simulink model "Output_Feedback_Teleoperation"  (Simulink 8.6)
settings: Solver=ode45  StartTime=0.0  StopTime=40  FixedStep=0.001  RelTol=1e-3
values from neighbouring files (symbols this model uses):
  c1 = 5    [Parameters.m]
  c2 = 5    [Parameters.m]
  c3 = 5    [Parameters.m]
  l1 = Prm(3)    [Coriolis.m]    (also in Inertia.m; P1.m; P2.m; Parameters.m = 0.4)
  l2 = Prm(4)    [Coriolis.m]    (also in Inertia.m; P1.m; P2.m; Parameters.m = 0.3)
  q_dot0 = [0;0]    [Parameters.m]
  q_hat0 = [0;0]    [Parameters.m]
  r_0 = 0    [Parameters.m]
  x_hat0 = [0;0]    [Parameters.m]
  xi_0 = [0;0]    [Parameters.m]
undefined symbols (not defined in the file or in its folder): cr, dm, ds, Kd, Kh, kl, kr, ml1, ml2, mr1, mr2, pl, pr, Pwall, ql_0, qr_0, sigbuilder_block
libraries: simulink x1
settings Model: Creator=TOSHIBA  LastModifiedBy=TOSHIBA
settings DataIOCC: SaveFormat=StructureWithTime  SignalLoggingSaveFormat=Dataset
settings OptimizationCC: ExpressionDepthLimit=128
settings DebuggingCC: UnderspecifiedInitializationDetection=Simplified  MergeDetectMultiDrivingBlocksExec=error  SolverPrmCheckMsg=none  FcnCallInpInsideContextMsg=EnableAllAsError  StateNameClashWarn=none
settings HardwareCC: ProdBitPerPointer=64  ProdLargestAtomicFloat=Float  ProdIntDivRoundTo=Zero  ProdEndianess=LittleEndian  ProdHWDeviceType=Specified
settings GRTTargetCC: GeneratePreprocessorConditionals=Use local settings  CombineOutputUpdateFcns=on  GRTInterface=off
settings ConfigComp: CovModelRefEnable=off

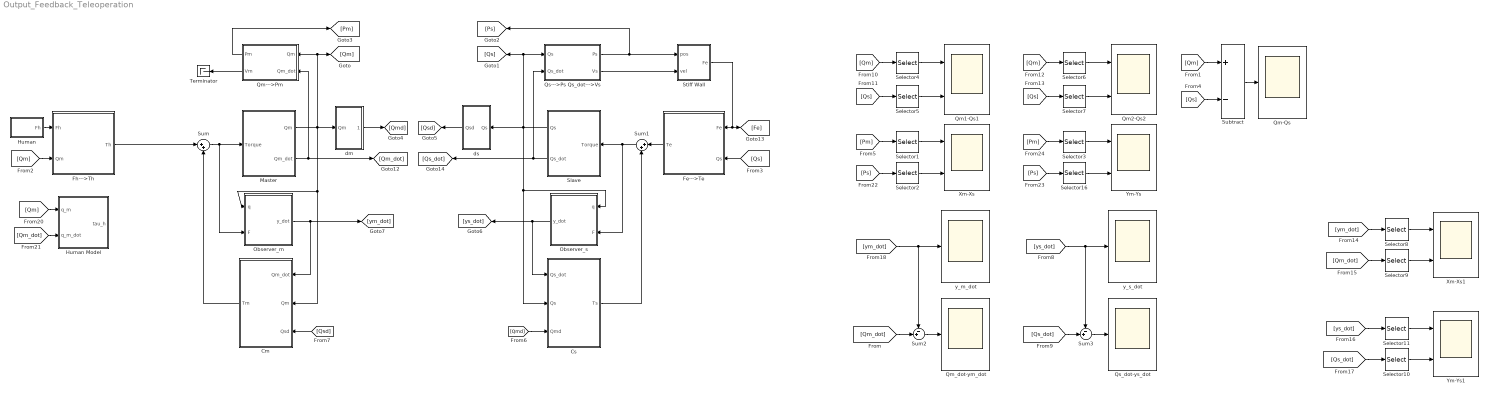
== system Output_Feedback_Teleoperation ==
  Cm : Subsystem
  Cs : Subsystem
  Fe--->Te : Subsystem
  Fh--->Th : Subsystem
  Human : Subsystem
  Human Model : Subsystem
  Master : Subsystem
  Observer_m : Subsystem
  Observer_s : Subsystem
  Qm--->Pm : Subsystem
  Qm-Qs : Scope
  Qm1-Qs1 : Scope  NumInputPorts=2
  Qm2-Qs2 : Scope  NumInputPorts=2
  Qm_dot-ym_dot : Scope
  Qs--->Ps Qs_dot--->Vs : Subsystem
  Qs_dot-ys_dot : Scope
  Selector{1..2,4..5,8..11} (8 alike) : Selector  InputPortWidth=2  IndexOptions=Index vector (dialog)  Indices=[1]  OutputSizes=1
  Selector{3,6..7,16} (4 alike) : Selector  InputPortWidth=2  IndexOptions=Index vector (dialog)  Indices=[2]  OutputSizes=1
  Slave : Subsystem
  Stiff Wall : Subsystem
  Subtract : Sum  Inputs=+-
  Sum : Sum  Inputs=|++
  Sum1 : Sum  Inputs=|++
  Sum2 : Sum  Inputs=-+|
  Sum3 : Sum  Inputs=-+|
  Terminator : Terminator
  Xm-Xs : Scope  NumInputPorts=2
  Xm-Xs1 : Scope  NumInputPorts=2
  Ym-Ys : Scope  NumInputPorts=2
  Ym-Ys1 : Scope  NumInputPorts=2
  dm : Subsystem
  ds : Subsystem
  y_m_dot : Scope
  y_s_dot : Scope
  wires:
  Fe--->Te/1(Te) -> Sum1/1
  Sum1/1 -> Observer_s/2(F), Slave/1(Torque)
  Sum/1 -> Observer_m/2(F), Master/1(Torque)
  Master/2(Qm_dot) -> Qm--->Pm/2(Qm_dot), [Qm_dot]
  Cm/1(Tm) -> Sum/2
  Slave/2(Qs_dot) -> [Qs_dot], Qs--->Ps Qs_dot--->Vs/2(Qs_dot)
  Cs/1(Ts) -> Sum1/2
  [Qs] -> Fe--->Te/2(Qs)
  Master/1(Qm) -> [Qm], Qm--->Pm/1(Qm), dm/1(Qm), Observer_m/1(q), Cm/2(Qm)
  Slave/1(Qs) -> Observer_s/1(q), Cs/2(Qs), ds/1(Qs), Qs--->Ps Qs_dot--->Vs/1(Qs), [Qs]
  [Qm] -> Fh--->Th/2(Qm)
  Qm--->Pm/1(Pm) -> [Pm]
  [Qmd] -> Cs/3(Qmd)
  ds/1(Qsd) -> [Qsd]
  dm/1(Qmd) -> [Qmd]
  [Qs] -> Selector5/1
  [Qm] -> Selector4/1
  Selector4/1 -> Qm1-Qs1/1
  Selector5/1 -> Qm1-Qs1/2
  [Qs] -> Selector7/1
  [Qm] -> Selector6/1
  Selector6/1 -> Qm2-Qs2/1
  Selector7/1 -> Qm2-Qs2/2
  Qs--->Ps Qs_dot--->Vs/2(Vs) -> Stiff Wall/2(vel)
  [Qsd] -> Cm/3(Qsd)
  Stiff Wall/1(Fe) -> [Fe], Fe--->Te/1(Fe)
  Qs--->Ps Qs_dot--->Vs/1(Ps) -> Stiff Wall/1(pos), [Ps]
  Qm--->Pm/2(Vm) -> Terminator/1
  Human/1(Fh) -> Fh--->Th/1(Fh)
  Observer_s/1(y_dot) -> Cs/1(Qs_dot), [ys_dot]
  [Qm] -> Human Model/1(q_m)
  [Qm_dot] -> Human Model/2(q_m_dot)
  [Qm] -> Subtract/1
  [Qs] -> Subtract/2
  Subtract/1 -> Qm-Qs/1
  [Pm] -> Selector1/1
  [Ps] -> Selector2/1
  Selector1/1 -> Xm-Xs/1
  Selector2/1 -> Xm-Xs/2
  [Pm] -> Selector3/1
  [Ps] -> Selector16/1
  Selector3/1 -> Ym-Ys/1
  Selector16/1 -> Ym-Ys/2
  [ym_dot] -> Sum2/1, y_m_dot/1
  [ys_dot] -> Sum3/1, y_s_dot/1
  Observer_m/1(y_dot) -> Cm/1(Qm_dot), [ym_dot]
  Sum2/1 -> Qm_dot-ym_dot/1
  [Qm_dot] -> Sum2/2
  [Qs_dot] -> Sum3/2
  Sum3/1 -> Qs_dot-ys_dot/1
  [ym_dot] -> Selector8/1
  [Qm_dot] -> Selector9/1
  Selector8/1 -> Xm-Xs1/1
  Selector9/1 -> Xm-Xs1/2
  [ys_dot] -> Selector11/1
  [Qs_dot] -> Selector10/1
  Selector11/1 -> Ym-Ys1/1
  Selector10/1 -> Ym-Ys1/2
  Fh--->Th/1(Th) -> Sum/1

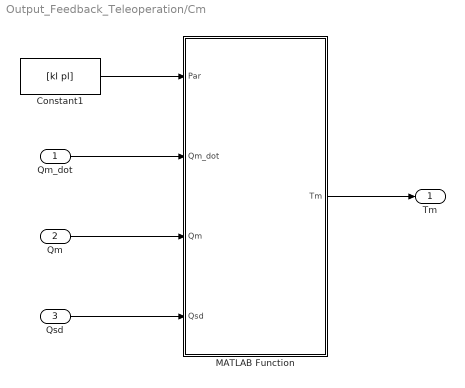
== system Output_Feedback_Teleoperation/Cm ==
  Qm_dot : Inport
  Qm : Inport  Port=2
  Qsd : Inport  Port=3
  Constant1 : Constant  Value=[kl pl]
  MATLAB Function : MATLAB Function  TreatAsAtomicUnit=on
  Tm : Outport
  wires:
  Qm_dot/1 -> MATLAB Function/2(Qm_dot)
  Qsd/1 -> MATLAB Function/4(Qsd)
  Constant1/1 -> MATLAB Function/1(Par)
  MATLAB Function/1(Tm) -> Tm/1
  Qm/1 -> MATLAB Function/3(Qm)

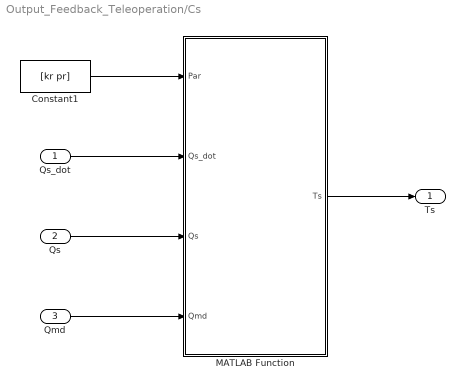
== system Output_Feedback_Teleoperation/Cs ==
  Qs_dot : Inport
  Qs : Inport  Port=2
  Qmd : Inport  Port=3
  Constant1 : Constant  Value=[kr pr]
  MATLAB Function : MATLAB Function  TreatAsAtomicUnit=on
  Ts : Outport
  wires:
  Qs_dot/1 -> MATLAB Function/2(Qs_dot)
  Qmd/1 -> MATLAB Function/4(Qmd)
  Constant1/1 -> MATLAB Function/1(Par)
  MATLAB Function/1(Ts) -> Ts/1
  Qs/1 -> MATLAB Function/3(Qs)

== system Output_Feedback_Teleoperation/Fe--->Te ==
  Fe : Inport
  Qs : Inport  Port=2
  Constant : Constant  Value=[l1,l2]
  MATLAB Function : MATLAB Function  TreatAsAtomicUnit=on
  Te : Outport
  wires:
  Qs/1 -> MATLAB Function/3(Q)
  Fe/1 -> MATLAB Function/2(F)
  MATLAB Function/1(T) -> Te/1
  Constant/1 -> MATLAB Function/1(Prm)

== system Output_Feedback_Teleoperation/Fh--->Th ==
  Fh : Inport
  Qm : Inport  Port=2
  Constant : Constant  Value=[l1,l2]
  MATLAB Function : MATLAB Function  TreatAsAtomicUnit=on
  Th : Outport
  wires:
  Fh/1 -> MATLAB Function/2(F)
  MATLAB Function/1(T) -> Th/1
  Qm/1 -> MATLAB Function/3(Q)
  Constant/1 -> MATLAB Function/1(Prm)

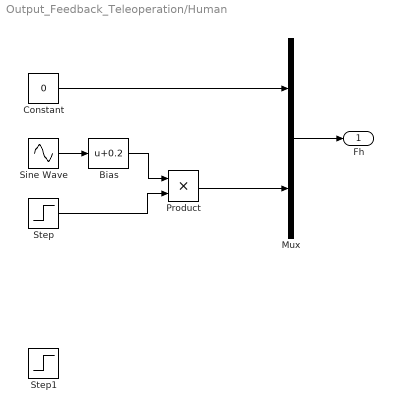
== system Output_Feedback_Teleoperation/Human ==
  Bias : Bias  Bias=0.2
  Constant : Constant  Value=0
  Mux : Mux  Inputs=2
  Product : Product
  Sine Wave : Sin  Frequency=pi/10  SampleTime=0
  Step : Step  Time=40  Before=1  After=0  SampleTime=0
  Step1 : Step  Time=0  After=0.5  SampleTime=0
  Fh : Outport
  wires:
  Mux/1 -> Fh/1
  Step/1 -> Product/2
  Bias/1 -> Product/1
  Sine Wave/1 -> Bias/1
  Product/1 -> Mux/2
  Constant/1 -> Mux/1

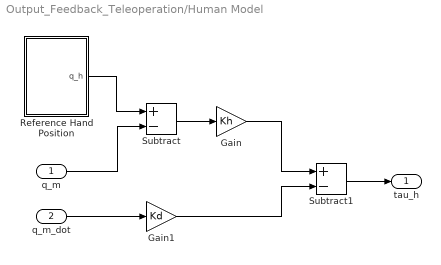
== system Output_Feedback_Teleoperation/Human Model ==
  q_m : Inport
  q_m_dot : Inport  Port=2
  Gain : Gain  Gain=Kh
  Gain1 : Gain  Gain=Kd
  Reference Hand Position : Subsystem
  Subtract : Sum  Inputs=+-
  Subtract1 : Sum  Inputs=+-
  tau_h : Outport
  wires:
  q_m_dot/1 -> Gain1/1
  q_m/1 -> Subtract/2
  Subtract1/1 -> tau_h/1
  Gain1/1 -> Subtract1/2
  Reference Hand Position/1(q_h) -> Subtract/1
  Gain/1 -> Subtract1/1
  Subtract/1 -> Gain/1

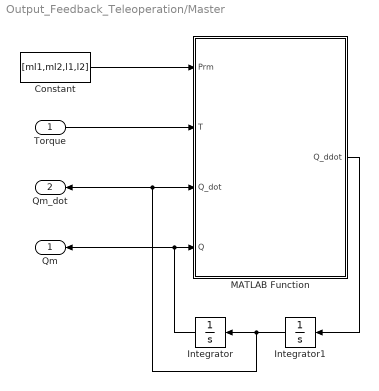
== system Output_Feedback_Teleoperation/Master ==
  Torque : Inport
  Constant : Constant  Value=[ml1,ml2,l1,l2]
  Integrator : Integrator  InitialCondition=ql_0
  Integrator1 : Integrator  InitialCondition=q_dot0
  MATLAB Function : MATLAB Function  TreatAsAtomicUnit=on
  Qm : Outport
  Qm_dot : Outport  Port=2
  wires:
  Torque/1 -> MATLAB Function/2(T)
  Constant/1 -> MATLAB Function/1(Prm)
  MATLAB Function/1(Q_ddot) -> Integrator1/1
  Integrator1/1 -> MATLAB Function/3(Q_dot), Qm_dot/1, Integrator/1
  Integrator/1 -> MATLAB Function/4(Q), Qm/1

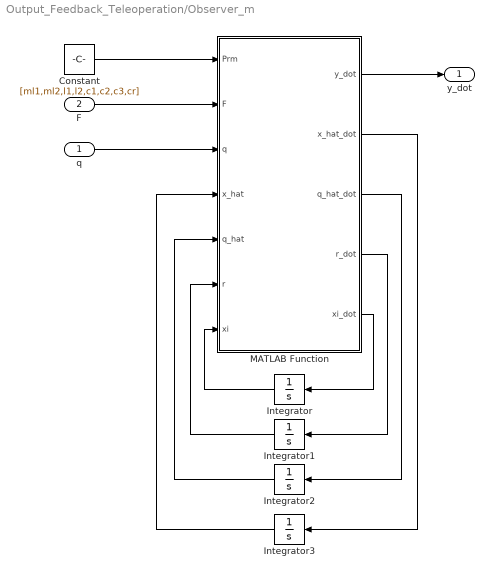
== system Output_Feedback_Teleoperation/Observer_m ==
  q : Inport
  F : Inport  Port=2
  Constant : Constant  Value=[ml1,ml2,l1,l2,c1,c2,c3,cr]
  Integrator : Integrator  InitialCondition=xi_0
  Integrator1 : Integrator  InitialCondition=r_0
  Integrator2 : Integrator  InitialCondition=q_hat0
  Integrator3 : Integrator  InitialCondition=x_hat0
  MATLAB Function : MATLAB Function  TreatAsAtomicUnit=on
  y_dot : Outport  PortDimensions=2
  wires:
  F/1 -> MATLAB Function/2(F)
  q/1 -> MATLAB Function/3(q)
  Constant/1 -> MATLAB Function/1(Prm)
  MATLAB Function/5(xi_dot) -> Integrator/1
  Integrator/1 -> MATLAB Function/7(xi)
  Integrator1/1 -> MATLAB Function/6(r)
  MATLAB Function/4(r_dot) -> Integrator1/1
  MATLAB Function/3(q_hat_dot) -> Integrator2/1
  Integrator2/1 -> MATLAB Function/5(q_hat)
  Integrator3/1 -> MATLAB Function/4(x_hat)
  MATLAB Function/2(x_hat_dot) -> Integrator3/1
  MATLAB Function/1(y_dot) -> y_dot/1

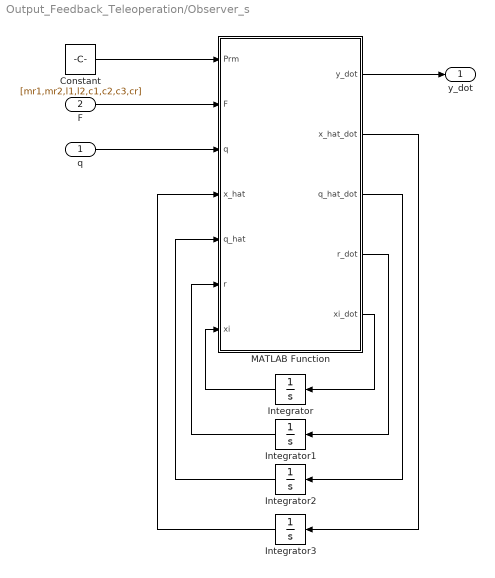
== system Output_Feedback_Teleoperation/Observer_s ==
  q : Inport
  F : Inport  Port=2
  Constant : Constant  Value=[mr1,mr2,l1,l2,c1,c2,c3,cr]
  Integrator : Integrator  InitialCondition=xi_0
  Integrator1 : Integrator  InitialCondition=r_0
  Integrator2 : Integrator  InitialCondition=q_hat0
  Integrator3 : Integrator  InitialCondition=x_hat0
  MATLAB Function : MATLAB Function  TreatAsAtomicUnit=on
  y_dot : Outport  PortDimensions=2
  wires:
  MATLAB Function/1(y_dot) -> y_dot/1
  MATLAB Function/2(x_hat_dot) -> Integrator3/1
  Integrator3/1 -> MATLAB Function/4(x_hat)
  Integrator2/1 -> MATLAB Function/5(q_hat)
  MATLAB Function/3(q_hat_dot) -> Integrator2/1
  MATLAB Function/4(r_dot) -> Integrator1/1
  Integrator1/1 -> MATLAB Function/6(r)
  Integrator/1 -> MATLAB Function/7(xi)
  MATLAB Function/5(xi_dot) -> Integrator/1
  Constant/1 -> MATLAB Function/1(Prm)
  q/1 -> MATLAB Function/3(q)
  F/1 -> MATLAB Function/2(F)

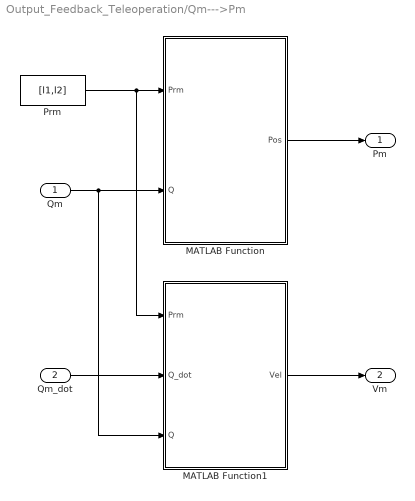
== system Output_Feedback_Teleoperation/Qm--->Pm ==
  Qm : Inport
  Qm_dot : Inport  Port=2
  MATLAB Function : MATLAB Function  TreatAsAtomicUnit=on
  MATLAB Function1 : MATLAB Function  TreatAsAtomicUnit=on
  Prm : Constant  Value=[l1,l2]
  Pm : Outport
  Vm : Outport  Port=2
  wires:
  MATLAB Function/1(Pos) -> Pm/1
  Qm/1 -> MATLAB Function1/3(Q), MATLAB Function/2(Q)
  Prm/1 -> MATLAB Function1/1(Prm), MATLAB Function/1(Prm)
  Qm_dot/1 -> MATLAB Function1/2(Q_dot)
  MATLAB Function1/1(Vel) -> Vm/1

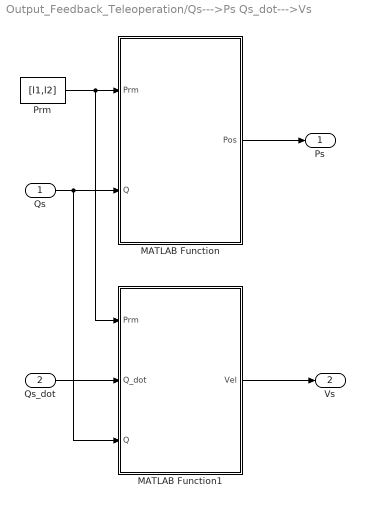
== system Output_Feedback_Teleoperation/Qs--->Ps Qs_dot--->Vs ==
  Qs : Inport
  Qs_dot : Inport  Port=2
  MATLAB Function : MATLAB Function  TreatAsAtomicUnit=on
  MATLAB Function1 : MATLAB Function  TreatAsAtomicUnit=on
  Prm : Constant  Value=[l1,l2]
  Ps : Outport
  Vs : Outport  Port=2
  wires:
  Qs/1 -> MATLAB Function1/3(Q), MATLAB Function/2(Q)
  MATLAB Function/1(Pos) -> Ps/1
  Prm/1 -> MATLAB Function1/1(Prm), MATLAB Function/1(Prm)
  Qs_dot/1 -> MATLAB Function1/2(Q_dot)
  MATLAB Function1/1(Vel) -> Vs/1

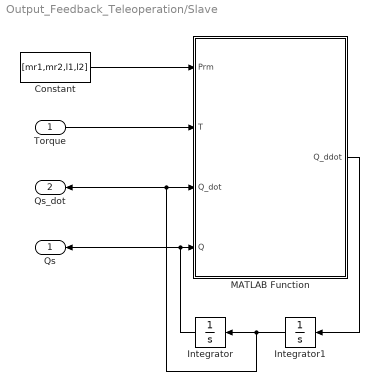
== system Output_Feedback_Teleoperation/Slave ==
  Torque : Inport
  Constant : Constant  Value=[mr1,mr2,l1,l2]
  Integrator : Integrator  InitialCondition=qr_0
  Integrator1 : Integrator  InitialCondition=q_dot0
  MATLAB Function : MATLAB Function  TreatAsAtomicUnit=on
  Qs : Outport
  Qs_dot : Outport  Port=2
  wires:
  Torque/1 -> MATLAB Function/2(T)
  Constant/1 -> MATLAB Function/1(Prm)
  MATLAB Function/1(Q_ddot) -> Integrator1/1
  Integrator1/1 -> Qs_dot/1, MATLAB Function/3(Q_dot), Integrator/1
  Integrator/1 -> Qs/1, MATLAB Function/4(Q)

== system Output_Feedback_Teleoperation/Stiff Wall ==
  pos : Inport
  vel : Inport  Port=2
  Constant : Constant  Value=Pwall
  Stiff Wall : MATLAB Function  TreatAsAtomicUnit=on
  Fe : Outport
  wires:
  vel/1 -> Stiff Wall/2(vel)
  pos/1 -> Stiff Wall/1(pos)
  Stiff Wall/1(Fe) -> Fe/1
  Constant/1 -> Stiff Wall/3(Pwall)

== system Output_Feedback_Teleoperation/dm ==
  Qm : Inport
  Constant : Constant  Value=dm
  Random Number : RandomNumber  Mean=0.2  Variance=0.003  Seed=0.3  SampleTime=0.1
  Uniform Random Number : UniformRandomNumber  Minimum=0  Maximum=dm  SampleTime=0.01
  Variable Time Delay : VariableTransportDelay  MaximumDelay=dm
  Qmd : Outport
  wires:
  Qm/1 -> Variable Time Delay/1
  Variable Time Delay/1 -> Qmd/1
  Uniform Random Number/1 -> Variable Time Delay/2

== system Output_Feedback_Teleoperation/ds ==
  Qs : Inport
  Constant : Constant  Value=ds
  Random Number : RandomNumber  Mean=0.4  Variance=0.004  Seed=0.5  SampleTime=0.1
  Uniform Random Number : UniformRandomNumber  Minimum=0  Maximum=ds  SampleTime=0.01
  Variable Time Delay : VariableTransportDelay  MaximumDelay=ds
  Qsd : Outport
  wires:
  Qs/1 -> Variable Time Delay/1
  Variable Time Delay/1 -> Qsd/1
  Uniform Random Number/1 -> Variable Time Delay/2

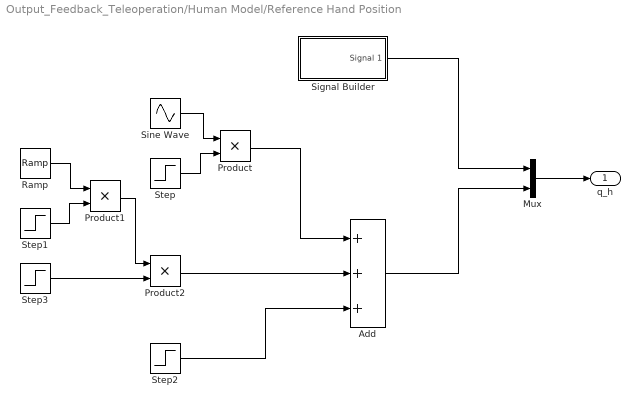
== system Output_Feedback_Teleoperation/Human Model/Reference Hand Position ==
  Add : Sum  Inputs=+++
  Mux : Mux  Inputs=2
  Product : Product
  Product1 : Product
  Product2 : Product
  Ramp : simulink/Sources/Ramp  slope=(1.6-1.6*sin(15*pi/16))/2  start=15  X0=1.6*sin(15*pi/16)
  Signal Builder : Subsystem  Tag=STV Subsys  LoadFcn=sigbuilder_block('load');  StartFcn=sigbuilder_block('start');  StopFcn=sigbuilder_block('stop');  ClipboardFcn=sigbuilder_block('clipboard');  mask(Sigbuilder block){}
      mask help: Simulink:masks:SigbuilderBlock_MD
      mask init:
      | if ~strcmp(get_param(bdroot(gcbh),'SimulationStatus'),'stopped') tuvar = sigbuilder_block('maskInit'); end
      settings: CopyFcn=sigbuilder_block('copy');  DeleteFcn=sigbuilder_block('delete');  ModelCloseFcn=sigbuilder_block('modelClose');  PreSaveFcn=sigbuilder_block('preSave');  PauseFcn=sigbuilder_block('pause');  ContinueFcn=sigbuilder_block('continue');  NameChangeFcn=sigbuilder_block('namechange');  OpenFcn=sigbuilder_block('open',[272.25 115.5 550.5 359.25 ]);  CloseFcn=sigbuilder_block('close');
      mask Display: plot(0, 0, 100, 100,[2, 2, 32, 32, 2], [68, 8, 8, 68, 68],[32, 2], [38, 38], [32, 19, 2],[53, 60, 44], [32, 17, 17, 2],[16, 16, 31, 31]);txt = getActiveGroup(gcbh);text(2, 100, txt,'verticalAlignment', 'top');
  Sine Wave : Sin  Amplitude=1.6  Frequency=pi/16  SampleTime=0
  Step : Step  Time=15  Before=1  After=0  SampleTime=0
  Step1 : Step  Time=17  Before=1  After=0  SampleTime=0
  Step2 : Step  Time=17  After=1.6  SampleTime=0
  Step3 : Step  Time=15  SampleTime=0
  q_h : Outport
  wires:
  Sine Wave/1 -> Product/1
  Step/1 -> Product/2
  Ramp/1 -> Product1/1
  Product/1 -> Add/1
  Step1/1 -> Product1/2
  Step2/1 -> Add/3
  Step3/1 -> Product2/2
  Product2/1 -> Add/2
  Product1/1 -> Product2/1
  Mux/1 -> q_h/1
  Signal Builder/1(Signal 1) -> Mux/1
  Add/1 -> Mux/2

== system Output_Feedback_Teleoperation/Human Model/Reference Hand Position/Signal Builder ==
  Demux : Demux  Tag=STV Demux  Outputs=1
  FromWs : FromWorkspace  Tag=STV FromWs  VariableName=tuvar  SampleTime=0  SigBuilderData=DataTag0  VnvData=DataTag1
      SigBuilderData=|
      | common.afterFinalStr = 'Extrapolate'
      | common.sampleTime = 0
      | dataSet.timeRange = [0 30]
      | dataSet.name = 'Group 1'
      | sbobj.Groups.Name = 'Group 1'
      | sbobj.Groups.Signals.Name = 'Signal 1'
      | sbobj.Groups.Signals.XData = [0 10 15 20 21.9 30]
      | sbobj.Groups.Signals.YData = [0 0 -1.1 -1.1 -1.1 -1.1]
      | sbobj.Groups.TimeRange = [0 30]
  Signal 1 : Outport  Tag=STV Outport
  wires:
  Demux/1 -> Signal 1/1
  FromWs/1 -> Demux/1

== matlab function Master/MATLAB Function ==
  data: Prm input double; Q_ddot output double; T input double; Q_dot input double; Q input double
function Q_ddot  = RobotArm_2DOF(Prm, T, Q_dot, Q)
%#codegen
g = 9.8;
m1 = Prm(1);
m2 = Prm(2);
l1 = Prm(3);
l2 = Prm(4);
q1 = Q(1);
q2 = Q(2);
q1_dot = Q_dot(1);
q2_dot = Q_dot(2);
M11 = m2*l2^2+(m1+m2)*l1^2+2*m2*l1*l2*cos(q2);
M12 = m2*l2^2+m2*l1*l2*cos(q2);
M21 = M12;
M22 = m2*l2^2;
M = [M11, M12; M21, M22];
C11 = -2*m2*l1*l2*sin(q2)*q2_dot;
C12 = -m2*l1*l2*sin(q2)*q2_dot;
C21 = m2*l1*l2*sin(q2)*q1_dot;
C22 = 0;
C = [C11, C12; C21, C22];
g1 = m2*g*l2*sin(q1+q2)+(m1+m2)*g*l1*sin(q1);
g2 = m2*g*l2*sin(q1+q2);
G = [g1; g2];
Q_ddot = M\(T-C*Q_dot);

== matlab function Stiff Wall/Stiff Wall ==
  data: pos input double; Fe output double; vel input double; Pwall input double
function Fe  = Envir(pos,vel,Pwall)
%#codegen
kWall = 10000;
bWall = 10;

if pos(2)>=Pwall
    Fk=[0; -(pos(2)-Pwall)*kWall];
    Fb=-bWall*[0;vel(2)];
    Fe=Fk+Fb;
    if Fe'*[0;1]>0
        Fe=[0;0];
    end
else
    Fe=zeros(2,1);
end

== matlab function Slave/MATLAB Function ==
  data: Prm input double; Q_ddot output double; T input double; Q_dot input double; Q input double
function Q_ddot  = RobotArm_2DOF(Prm, T, Q_dot, Q)
%#codegen
g = 9.8;
m1 = Prm(1);
m2 = Prm(2);
l1 = Prm(3);
l2 = Prm(4);
q1 = Q(1);
q2 = Q(2);
q1_dot = Q_dot(1);
q2_dot = Q_dot(2);
M11 = m2*l2^2+(m1+m2)*l1^2+2*m2*l1*l2*cos(q2);
M12 = m2*l2^2+m2*l1*l2*cos(q2);
M21 = M12;
M22 = m2*l2^2;
M = [M11, M12; M21, M22];
C11 = -2*m2*l1*l2*sin(q2)*q2_dot;
C12 = -m2*l1*l2*sin(q2)*q2_dot;
C21 = m2*l1*l2*sin(q2)*q1_dot;
C22 = 0;
C = [C11, C12; C21, C22];
g1 = m2*g*l2*sin(q1+q2)+(m1+m2)*g*l1*sin(q1);
g2 = m2*g*l2*sin(q1+q2);
G = [g1; g2];
Q_ddot = M\(T-C*Q_dot);

== matlab function Qm--->Pm/MATLAB Function ==
  data: Prm input double; Pos output double; Q input double
function Pos = ForwardKinematics(Prm, Q)
%#codegen
l1 = Prm(1);
l2 = Prm(2);
q1 = Q(1);
q2 = Q(2);
x = l1*cos(q1)+l2*cos(q1+q2);
y = l1*sin(q1)+l2*sin(q1+q2);
Pos = [x; y];

== matlab function Qs--->Ps Qs_dot--->Vs/MATLAB Function ==
  data: Prm input double; Pos output double; Q input double
function Pos = ForwardKinematics(Prm, Q)
%#codegen
l1 = Prm(1);
l2 = Prm(2);
q1 = Q(1);
q2 = Q(2);
x = l1*cos(q1)+l2*cos(q1+q2);
y = l1*sin(q1)+l2*sin(q1+q2);
Pos = [x; y];

== matlab function Fh--->Th/MATLAB Function ==
  data: Prm input double; T output double; F input double; Q input double
function T = Force_to_Torque(Prm, F, Q)
%#codegen
l1 = Prm(1);
l2 = Prm(2);
q1 = Q(1);
q2 = Q(2);
J11 = -l1*sin(q1)-l2*sin(q1+q2);
J12 = -l2*sin(q1+q2);
J21 = l1*cos(q1)+l2*cos(q1+q2);
J22 = l2*cos(q1+q2);
J = [J11, J12; J21, J22];
T = J'*F;

== matlab function Fe--->Te/MATLAB Function ==
  data: Prm input double; T output double; F input double; Q input double
function T = Force_to_Torque(Prm, F, Q)
%#codegen
l1 = Prm(1);
l2 = Prm(2);
q1 = Q(1);
q2 = Q(2);
J11 = -l1*sin(q1)-l2*sin(q1+q2);
J12 = -l2*sin(q1+q2);
J21 = l1*cos(q1)+l2*cos(q1+q2);
J22 = l2*cos(q1+q2);
J = [J11, J12; J21, J22];
T = J'*F;

== matlab function Cs/MATLAB Function ==
  data: Par input double; Ts output double; Qs_dot input double; Qs input double; Qmd input double
function Ts = fcn(Par,Qs_dot,Qs,Qmd)
%#codegen

ks = Par(1);
ps = Par(2);

Ks = ks*eye(2);
Ps = ps*eye(2);

Ts = -Ps*(Qs-Qmd)-Ks*Qs_dot;

== matlab function Qm--->Pm/MATLAB Function1 ==
  data: Prm input double; Vel output double; Q_dot input double; Q input double
function Vel = Velocity_Jacobian(Prm, Q_dot, Q)
%#codegen
l1 = Prm(1);
l2 = Prm(2);
q1 = Q(1);
q2 = Q(2);
J11 = -l1*sin(q1)-l2*sin(q1+q2);
J12 = -l2*sin(q1+q2);
J21 = l1*cos(q1)+l2*cos(q1+q2);
J22 = l2*cos(q1+q2);
J = [J11, J12; J21, J22];
Vel=J*Q_dot;

== matlab function Qs--->Ps Qs_dot--->Vs/MATLAB Function1 ==
  data: Prm input double; Vel output double; Q_dot input double; Q input double
function Vel = Velocity_Jacobian(Prm, Q_dot, Q)
%#codegen
l1 = Prm(1);
l2 = Prm(2);
q1 = Q(1);
q2 = Q(2);
J11 = -l1*sin(q1)-l2*sin(q1+q2);
J12 = -l2*sin(q1+q2);
J21 = l1*cos(q1)+l2*cos(q1+q2);
J22 = l2*cos(q1+q2);
J = [J11, J12; J21, J22];
Vel=J*Q_dot;

== matlab function Cm/MATLAB Function ==
  data: Par input double; Tm output double; Qm_dot input double; Qm input double; Qsd input double
function Tm  = fcn(Par,Qm_dot,Qm,Qsd)
%#codegen

km = Par(1);
pm = Par(2);

Km = km*eye(2);
Pm = pm*eye(2);

Tm = -Pm*(Qm-Qsd)-Km*Qm_dot;

== matlab function Observer_m/MATLAB Function ==
  data: Prm input double; F input double; q input double; x_hat input double; q_hat input double; r input double; xi input double; y_dot output double; x_hat_dot output double; q_hat_dot output double; r_dot output double; xi_dot output double
function [y_dot, x_hat_dot, q_hat_dot, r_dot, xi_dot] = Observer(Prm, F, q, x_hat, q_hat, r, xi)

c1 = Prm(5);
c2 = Prm(6);
c3 = Prm(7);
cr = Prm(8);

psi3 = r^2*norm(L(Prm,q))^2+c1;
% psi3 =c1;

k = 4*(1+psi3);

beta = H(Prm,k,q_hat,x_hat)*q;
ex = x_hat-(xi+beta);
eq = q_hat-q;

if norm(eq)~=0
    Dq_bar = norm(Delta_q(Prm,k,q,q_hat,x_hat))/norm(eq);
else
    Dq_bar = 0;
end

if norm(ex)~=0
    Dx_bar = norm(Delta_x(Prm,q,ex))/norm(ex);
else
    Dx_bar = 0;
end

psi4 = norm(L(Prm,q))^2+0.25*r^2/(1+psi3)*norm(L(Prm,q))^2*Dx_bar^2+c2;
psi5 = 0.25*r^2/(1+psi3)*norm(L(Prm,q))^2*norm(Dq_bar)^2+c3;

x_hat_dot = F+S(Prm,q,xi+beta)*(xi+beta)-0.5*r^2*norm(H(Prm,k,q_hat,x_hat))^2*norm(L(Prm,q))^2*ex-psi4*ex;
q_hat_dot = L(Prm,q)*(xi+beta)-0.5*r^2*norm(L(Prm,q))^2*eq-psi5*eq;
r_dot = -0.25*k*(r-cr)+r/k*(norm(Delta_x(Prm,q,ex)*L(Prm,q))^2+norm(Delta_q(Prm,k,q,q_hat,x_hat))^2);
xi_dot = F-partial_beta_qhat(Prm,k,q,q_hat,x_hat)*q_hat_dot-partial_beta_xhat(Prm,q,q_hat)*x_hat_dot+S(Prm,q,xi+beta)*(xi+beta)-H(Prm,k,q_hat,x_hat)*L(Prm,q)*(xi+beta);

y_dot = L(Prm,q)*(xi+beta);

== matlab function Observer_s/MATLAB Function ==
  data: Prm input double; F input double; q input double; x_hat input double; q_hat input double; r input double; xi input double; y_dot output double; x_hat_dot output double; q_hat_dot output double; r_dot output double; xi_dot output double
function [y_dot, x_hat_dot, q_hat_dot, r_dot, xi_dot] = Observer(Prm, F, q, x_hat, q_hat, r, xi)

c1 = Prm(5);
c2 = Prm(6);
c3 = Prm(7);
cr = Prm(8);

% psi3 = r^2*norm(L(Prm,q))^2+c1;
 psi3 = c1;

k = 4*(1+psi3);

beta = H(Prm,k,q_hat,x_hat)*q;
ex = x_hat-(xi+beta);
eq = q_hat-q;

if norm(eq)~=0
    Dq_bar = norm(Delta_q(Prm,k,q,q_hat,x_hat))/norm(eq);
else
    Dq_bar = 0;
end

if norm(ex)~=0
    Dx_bar = norm(Delta_x(Prm,q,ex))/norm(ex);
else
    Dx_bar = 0;
end

psi4 = norm(L(Prm,q))^2+0.25*r^2/(1+psi3)*norm(L(Prm,q))^2*Dx_bar^2+c2;
psi5 = 0.25*r^2/(1+psi3)*norm(L(Prm,q))^2*norm(Dq_bar)^2+c3;

x_hat_dot = F+S(Prm,q,xi+beta)*(xi+beta)-0.5*r^2*norm(H(Prm,k,q_hat,x_hat))^2*norm(L(Prm,q))^2*ex-psi4*ex;
q_hat_dot = L(Prm,q)*(xi+beta)-0.5*r^2*norm(L(Prm,q))^2*eq-psi5*eq;
r_dot = -0.25*k*(r-cr)+r/k*(norm(Delta_x(Prm,q,ex)*L(Prm,q))^2+norm(Delta_q(Prm,k,q,q_hat,x_hat))^2);
xi_dot = F-partial_beta_qhat(Prm,k,q,q_hat,x_hat)*q_hat_dot-partial_beta_xhat(Prm,q,q_hat)*x_hat_dot+S(Prm,q,xi+beta)*(xi+beta)-H(Prm,k,q_hat,x_hat)*L(Prm,q)*(xi+beta);

y_dot = L(Prm,q)*(xi+beta);
